simulink model "chap6_2sim"  (R2015a)
settings: Solver=ode45  StartTime=0.0  StopTime=30  FixedStep=0.01  RelTol=1e-3
settings Model: Creator=Masoud  LastModifiedBy=Masoud

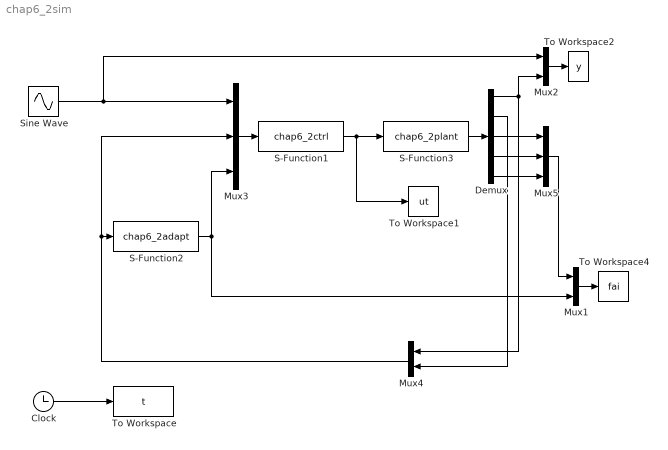
== system chap6_2sim ==
  Clock : Clock
  Demux : Demux  Outputs=5
  Mux1 : Mux  Inputs=2
  Mux2 : Mux  Inputs=2
  Mux3 : Mux  Inputs=3
  Mux4 : Mux  Inputs=2
  Mux5 : Mux  Inputs=3
  S-Function1 : S-Function  FunctionName=chap6_2ctrl  SFunctionModules='chap6_2ctrl'
  S-Function2 : S-Function  FunctionName=chap6_2adapt  SFunctionModules='chap6_2adapt'
  S-Function3 : S-Function  FunctionName=chap6_2plant  SFunctionModules='chap6_2plant'
  Sine Wave : Sin  Amplitude=0.1  SampleTime=0
  To Workspace : ToWorkspace  VariableName=t  SampleTime=-1
  To Workspace1 : ToWorkspace  VariableName=ut  SampleTime=-1
  To Workspace2 : ToWorkspace  VariableName=y  SampleTime=-1
  To Workspace4 : ToWorkspace  VariableName=fai  SampleTime=-1
  wires:
  Clock/1 -> To Workspace/1
  Mux2/1 -> To Workspace2/1
  S-Function2/1 -> Mux1/2, Mux3/3
  S-Function1/1 -> S-Function3/1, To Workspace1/1
  Sine Wave/1 -> Mux3/1, Mux2/1
  Mux4/1 -> Mux3/2, S-Function2/1
  Mux3/1 -> S-Function1/1
  S-Function3/1 -> Demux/1
  Demux/1 -> Mux4/1, Mux2/2
  Demux/2 -> Mux4/2
  Mux1/1 -> To Workspace4/1
  Demux/3 -> Mux5/1
  Demux/4 -> Mux5/2
  Demux/5 -> Mux5/3
  Mux5/1 -> Mux1/1
